simulink subsystem "battery_segment"  (R2021a)
settings: Solver=VariableStepAuto  StartTime=0.0  StopTime=10.0  RelTol=1e-3
libraries: fl_lib x5, nesl_utility x1
settings Model: Creator=Carlo Edoardo  LastModifiedBy=Carlo Edoardo

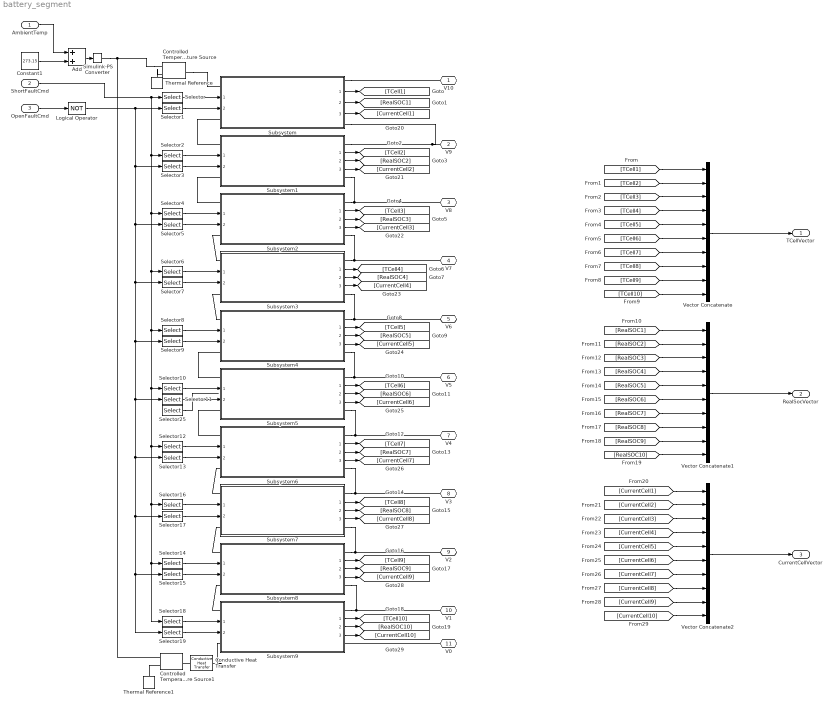
== system battery_segment ==
  AmbientTemp : Inport
  ShortFaultCmd : Inport  Port=2
  OpenFaultCmd : Inport  Port=3  OutDataTypeStr=boolean
  Add : Sum
  Conductive Heat Transfer : fl_lib/Thermal/Thermal Elements/Conductive Heat Transfer  area=LowerSegmentConductiveArea m^2  thickness=LowerSegmentConductiveThickness mm  th_cond=LowerSegmentConductiveThermConduct W/(m*K)  T_specify=off  T_priority=None  T=0 K  T_nominal_specify=off  T_nominal_unit=K  T_nominal_value=1  Q_specify=off  Q_priority=None  Q=0 W  Q_nominal_specify=off  Q_nominal_unit=W  Q_nominal_value=1
  Constant1 : Constant  Value=273.15
  Controlled Temperature Source : fl_lib/Thermal/Thermal Sources/Controlled Temperature Source
  Controlled Temperature Source1 : fl_lib/Thermal/Thermal Sources/Controlled Temperature Source
  Logical Operator : Logic  Operator=NOT  AllPortsSameDT=off  OutDataTypeStr=boolean
  Selector : Selector  InputPortWidth=10  IndexOptions=Index vector (dialog)  Indices=1  OutputSizes=1
  Selector1 : Selector  InputPortWidth=10  IndexOptions=Index vector (dialog)  Indices=1  OutputSizes=1
  Selector10 : Selector  InputPortWidth=10  IndexOptions=Index vector (dialog)  Indices=6  OutputSizes=1
  Selector11 : Selector  InputPortWidth=10  IndexOptions=Index vector (dialog)  Indices=6  OutputSizes=1
  Selector12 : Selector  InputPortWidth=10  IndexOptions=Index vector (dialog)  Indices=7  OutputSizes=1
  Selector13 : Selector  InputPortWidth=10  IndexOptions=Index vector (dialog)  Indices=7  OutputSizes=1
  Selector14 : Selector  InputPortWidth=10  IndexOptions=Index vector (dialog)  Indices=9  OutputSizes=1
  Selector15 : Selector  InputPortWidth=10  IndexOptions=Index vector (dialog)  Indices=9  OutputSizes=1
  Selector16 : Selector  InputPortWidth=10  IndexOptions=Index vector (dialog)  Indices=8  OutputSizes=1
  Selector17 : Selector  InputPortWidth=10  IndexOptions=Index vector (dialog)  Indices=8  OutputSizes=1
  Selector18 : Selector  InputPortWidth=10  IndexOptions=Index vector (dialog)  Indices=10  OutputSizes=1
  Selector19 : Selector  InputPortWidth=10  IndexOptions=Index vector (dialog)  Indices=10  OutputSizes=1
  Selector2 : Selector  InputPortWidth=10  IndexOptions=Index vector (dialog)  Indices=2  OutputSizes=1
  Selector25 : Selector  InputPortWidth=10  IndexOptions=Index vector (dialog)  Indices=6  OutputSizes=1
  Selector3 : Selector  InputPortWidth=10  IndexOptions=Index vector (dialog)  Indices=2  OutputSizes=1
  Selector4 : Selector  InputPortWidth=10  IndexOptions=Index vector (dialog)  Indices=3  OutputSizes=1
  Selector5 : Selector  InputPortWidth=10  IndexOptions=Index vector (dialog)  Indices=3  OutputSizes=1
  Selector6 : Selector  InputPortWidth=10  IndexOptions=Index vector (dialog)  Indices=4  OutputSizes=1
  Selector7 : Selector  InputPortWidth=10  IndexOptions=Index vector (dialog)  Indices=4  OutputSizes=1
  Selector8 : Selector  InputPortWidth=10  IndexOptions=Index vector (dialog)  Indices=5  OutputSizes=1
  Selector9 : Selector  InputPortWidth=10  IndexOptions=Index vector (dialog)  Indices=5  OutputSizes=1
  Simulink-PS Converter : nesl_utility/Simulink-PS Converter  PhysicalDomain=network_engine_domain  SubClassName=ps_input  LeftPortType=input  RightPortType=output  PseudoPeriodic=off  Frequencies=[]  NoiseDistribution=none  NoiseParameters=[]  Unit=1  AffineConversion=off  FilteringAndDerivatives=provide  SimscapeFilterOrder=1  InputFilterTimeConstant=0.001  UdotUserProvided=0
      settings: SourceProductBaseCode=PW,SS
  Subsystem{,1..9} (10 alike) : Subsystem  ReferencedSubsystem=single_cell
      settings: PortSchema="{\"entries\":[{\"content\":{\"sides\":[{\"content\":{\"connectorIds\":[\"LConn1\",\"In1\",\"In2\",\"LConn2\"]},\"type\":\"ConnectorPlacement.EquallySpacedRectSide\",\"uuid\":\"8db1a100-dcc8-40d2-b104-496cf3689302\"},{\"content\":{\"connectorIds\":[\"RConn1\",\"Out1\",\"Out2\",\"Out3\",\"RConn2\"],\"side\":\"RIGHT\"},\"type\":\"ConnectorPlacement.EquallySpacedRectSide\",\"uuid\":\"820dccfa-364b-4592-b089-b9752bf72c70\"},{\"content\":{\"connectorIds\":[],\"side\":\"TOP\"},\"type\":\"ConnectorPlacement.EquallySpacedRectSide\",\"uuid\":\"a43b9d45-4457-4465-8771-f1b49989aeb9\"}]},\"type\":\"ConnectorPlacement.EquallySpacedConnector\",\"uuid\":\"19838d43-a1b6-4b3f-844a-5adb2152d4ee\"}],\"packageUris\":[\"http://schema.mathworks.com/mf0/Connector/R2020b\"],\"version\":\"1.0\"}"
  Thermal Reference : fl_lib/Thermal/Thermal Elements/Thermal Reference
  Thermal Reference1 : fl_lib/Thermal/Thermal Elements/Thermal Reference
  Vector Concatenate : Concatenate  NumInputs=10
  Vector Concatenate1 : Concatenate  NumInputs=10
  Vector Concatenate2 : Concatenate  NumInputs=10
  V10 : PMIOPort  Side=Right
  V9 : PMIOPort  Port=2  Side=Right
  V8 : PMIOPort  Port=3  Side=Right
  V7 : PMIOPort  Port=4  Side=Right
  V6 : PMIOPort  Port=5  Side=Right
  V5 : PMIOPort  Port=6  Side=Right
  V4 : PMIOPort  Port=7  Side=Right
  V3 : PMIOPort  Port=8  Side=Right
  V2 : PMIOPort  Port=9  Side=Right
  V1 : PMIOPort  Port=10  Side=Right
  V0 : PMIOPort  Port=11  Side=Right
  TCellVector : Outport
  RealSocVector : Outport  Port=2
  CurrentCellVector : Outport  Port=3
  wires:
  [CurrentCell10] -> Vector Concatenate2/10
  [CurrentCell9] -> Vector Concatenate2/9
  [CurrentCell8] -> Vector Concatenate2/8
  [CurrentCell7] -> Vector Concatenate2/7
  [CurrentCell6] -> Vector Concatenate2/6
  [CurrentCell5] -> Vector Concatenate2/5
  [CurrentCell4] -> Vector Concatenate2/4
  [CurrentCell3] -> Vector Concatenate2/3
  [CurrentCell2] -> Vector Concatenate2/2
  [CurrentCell1] -> Vector Concatenate2/1
  Vector Concatenate2/1 -> CurrentCellVector/1
  Subsystem9/3 -> [CurrentCell10]
  Subsystem8/3 -> [CurrentCell9]
  Subsystem7/3 -> [CurrentCell8]
  Subsystem6/3 -> [CurrentCell7]
  Subsystem5/3 -> [CurrentCell6]
  Subsystem5/2 -> [RealSOC6]
  Subsystem4/3 -> [CurrentCell5]
  Subsystem3/3 -> [CurrentCell4]
  Subsystem2/3 -> [CurrentCell3]
  Subsystem1/3 -> [CurrentCell2]
  Subsystem/3 -> [CurrentCell1]
  [RealSOC10] -> Vector Concatenate1/10
  [RealSOC9] -> Vector Concatenate1/9
  [RealSOC8] -> Vector Concatenate1/8
  [RealSOC7] -> Vector Concatenate1/7
  [RealSOC6] -> Vector Concatenate1/6
  [RealSOC5] -> Vector Concatenate1/5
  [RealSOC4] -> Vector Concatenate1/4
  [RealSOC3] -> Vector Concatenate1/3
  [RealSOC2] -> Vector Concatenate1/2
  [RealSOC1] -> Vector Concatenate1/1
  Vector Concatenate1/1 -> RealSocVector/1
  [TCell10] -> Vector Concatenate/10
  [TCell9] -> Vector Concatenate/9
  [TCell8] -> Vector Concatenate/8
  [TCell7] -> Vector Concatenate/7
  [TCell6] -> Vector Concatenate/6
  [TCell5] -> Vector Concatenate/5
  [TCell4] -> Vector Concatenate/4
  [TCell3] -> Vector Concatenate/3
  [TCell2] -> Vector Concatenate/2
  [TCell1] -> Vector Concatenate/1
  Subsystem9/2 -> [RealSOC10]
  Subsystem9/1 -> [TCell10]
  Subsystem8/2 -> [RealSOC9]
  Subsystem8/1 -> [TCell9]
  Subsystem7/2 -> [RealSOC8]
  Subsystem7/1 -> [TCell8]
  Subsystem6/2 -> [RealSOC7]
  Subsystem6/1 -> [TCell7]
  Subsystem5/1 -> [TCell6]
  Subsystem4/2 -> [RealSOC5]
  Subsystem4/1 -> [TCell5]
  Subsystem3/2 -> [RealSOC4]
  Subsystem3/1 -> [TCell4]
  Subsystem2/2 -> [RealSOC3]
  Subsystem2/1 -> [TCell3]
  Subsystem1/2 -> [RealSOC2]
  Subsystem1/1 -> [TCell2]
  Subsystem/2 -> [RealSOC1]
  Subsystem/1 -> [TCell1]
  Selector25/1 -> ?
  AmbientTemp/1 -> Add/1
  Add/1 -> Simulink-PS Converter/1
  Constant1/1 -> Add/2
  Logical Operator/1 -> Selector19/1, Selector15/1, Selector17/1, Selector13/1, Selector11/1, Selector9/1, Selector7/1, Selector5/1, Selector3/1, Selector1/1
  Selector16/1 -> Subsystem7/1
  Selector13/1 -> Subsystem6/2
  Selector9/1 -> Subsystem4/2
  Selector5/1 -> Subsystem2/2
  Selector18/1 -> Subsystem9/1
  Selector17/1 -> Subsystem7/2
  Selector/1 -> Subsystem/1
  Selector2/1 -> Subsystem1/1
  Selector6/1 -> Subsystem3/1
  Selector8/1 -> Subsystem4/1
  Selector14/1 -> Subsystem8/1
  Selector4/1 -> Subsystem2/1
  Selector1/1 -> Subsystem/2
  Selector10/1 -> Subsystem5/1
  Selector11/1 -> Subsystem5/2
  Selector19/1 -> Subsystem9/2
  Selector15/1 -> Subsystem8/2
  ShortFaultCmd/1 -> Selector2/1, Selector4/1, Selector18/1, Selector14/1, Selector16/1, Selector12/1, Selector10/1, Selector8/1, Selector6/1, Selector/1
  Selector7/1 -> Subsystem3/2
  Selector12/1 -> Subsystem6/1
  Selector3/1 -> Subsystem1/2
  OpenFaultCmd/1 -> Logical Operator/1
  Vector Concatenate/1 -> TCellVector/1
  connections:
  Subsystem9/RConn1 -- V1/RConn1 -- Subsystem8/RConn2
  Subsystem8/RConn1 -- V2/RConn1 -- Subsystem7/RConn2
  Subsystem7/RConn1 -- V3/RConn1 -- Subsystem6/RConn2
  Subsystem6/RConn1 -- Subsystem5/RConn2 -- V4/RConn1
  Subsystem5/RConn1 -- Subsystem4/RConn2 -- V5/RConn1
  Subsystem4/RConn1 -- Subsystem3/RConn2 -- V6/RConn1
  Subsystem3/RConn1 -- Subsystem2/RConn2 -- V7/RConn1
  Subsystem2/RConn1 -- Subsystem1/RConn2 -- V8/RConn1
  Subsystem1/RConn1 -- V9/RConn1 -- Subsystem/RConn2
  Controlled Temperature Source/RConn1 -- Simulink-PS Converter/RConn1 -- Controlled Temperature Source1/RConn1
  Conductive Heat Transfer/RConn1 -- Subsystem9/LConn2
  Conductive Heat Transfer/LConn1 -- Controlled Temperature Source1/LConn1
  Controlled Temperature Source1/RConn2 -- Thermal Reference1/LConn1
  Subsystem/RConn1 -- V10/RConn1
  Subsystem1/LConn2 -- Subsystem2/LConn1
  Subsystem2/LConn2 -- Subsystem3/LConn1
  Subsystem3/LConn2 -- Subsystem4/LConn1
  Subsystem4/LConn2 -- Subsystem5/LConn1
  Subsystem6/LConn1 -- Subsystem5/LConn2
  Subsystem7/LConn1 -- Subsystem6/LConn2
  Subsystem8/LConn1 -- Subsystem7/LConn2
  Subsystem9/LConn1 -- Subsystem8/LConn2
  Subsystem1/LConn1 -- Subsystem/LConn2
  Controlled Temperature Source/LConn1 -- Subsystem/LConn1
  Thermal Reference/LConn1 -- Controlled Temperature Source/RConn2
  V0/RConn1 -- Subsystem9/RConn2
